simulink model "system_2022 [23-03-03]"  (R2022a)
settings: Solver=FixedStepAuto  StartTime=0.0  StopTime=30  FixedStep=0.05  MinStep=0.01  RelTol=1e-3  EnableMultiTasking=on
libraries: mbedblockslib x24, simulink x6, hdlsllib x6, slpidlib x3
(part 1 of 3)
settings Model: ExtModeTrigDuration=10  Creator=MATLAB  LastModifiedBy=FUGAZI
settings SolverCC: ZeroCrossControl=DisableAll  AutoInsertRateTranBlk=on
settings OptimizationCC: EnhancedBackFolding=on  PassReuseOutputArgsAs=Individual arguments  ZeroExternalMemoryAtStartup=off  ZeroInternalMemoryAtStartup=off  MaxStackSize=64  OptimizeBlockOrder=speed  DifferentSizesBufferReuse=on  OptimizationCustomize=off  EfficientTunableParamExpr=on
settings DebuggingCC: MultiTaskDSMMsg=none  ParameterTunabilityLossMsg=error
settings HardwareCC: ProdBitPerPointer=32  ProdBitPerSizeT=32  ProdBitPerPtrDiffT=32  ProdLargestAtomicInteger=Long  ProdLargestAtomicFloat=Double  ProdWordSize=32  ProdLongLongMode=on  ProdHWDeviceType=ARM Compatible->ARM Cortex
settings SFSimCC: MATLABDynamicMemAlloc=off
settings RTWCC: SystemTargetFile=ert.tlc  HardwareBoard=STM32 Nucleo L476RG  TemplateMakefile=ert_default_tmf  Toolchain=GNU Tools for ARM Embedded Processors
settings CodeAppCC: ForceParamTrailComments=on  IgnoreCustomStorageClasses=off  OperatorAnnotations=on  SimulinkDataObjDesc=on  SFDataObjDesc=on  InsertBlockDesc=on
settings ERTTargetCC: SupportContinuousTime=on  ExtModeTransport=3  ExtModeStaticAlloc=on  ExtModeStaticAllocSize=2000  ExtModeMexFile=ext_xcp  ExtModeIntrfLevel=Level2 - Open

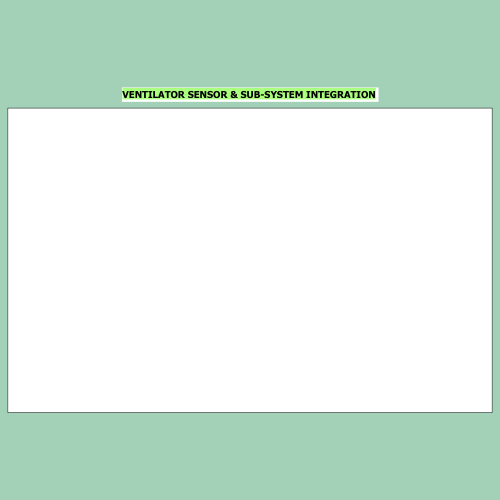
[thumbnail: Simulink's stored preview of the top-level diagram]
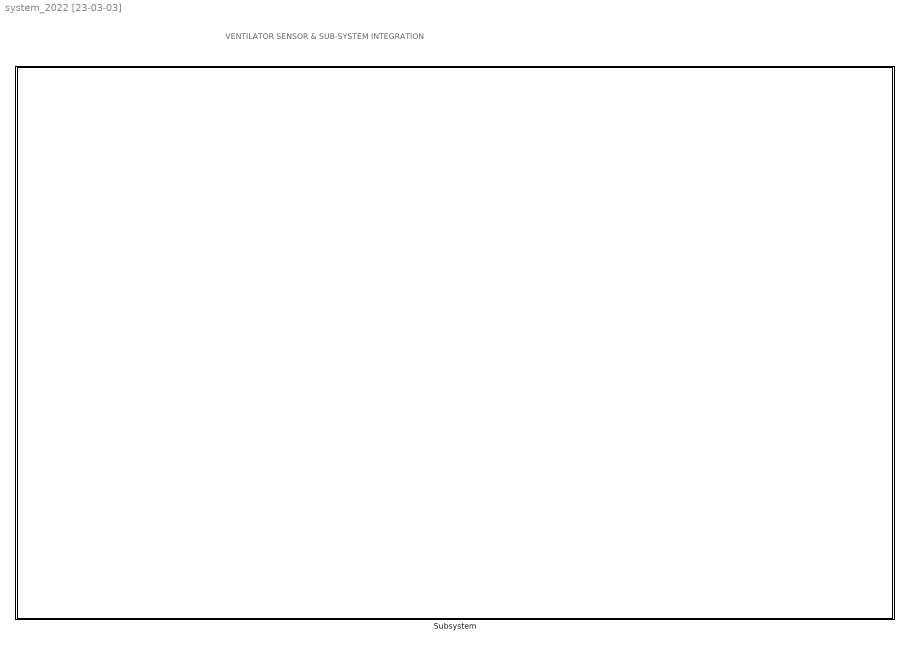
== system system_2022 [23-03-03] ==
  note: VENTILATOR SENSOR & SUB-SYSTEM INTEGRATION
  Subsystem : Subsystem

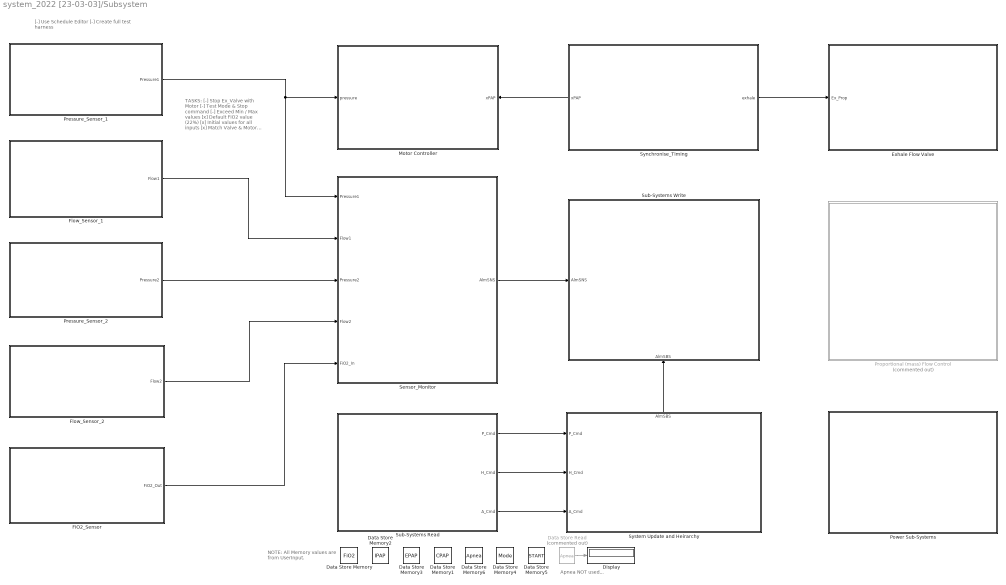
== system system_2022 [23-03-03]/Subsystem ==
  note: Apnea NOT used...
  note: TASKS:
      | [-] Stop Ex_Valve with Motor
      | [-] Test Mode & Stop command
      | [-] Exceed Min / Max values
      | [x] Default FiO2 value (22%)
      | [x] Initial values for all inputs
      | [x] Match Valve & Motor timing
      | [x] Start/Stop bit activate
      | [x] CPAP / BiPAP Mode select
      | [x] Initial CPAP value at boot
  note: [-] Use Schedule Editor
      | [-] Create full test harness
  note: NOTE: All Memory values
      | are from UserInput.
  Data Store Memory : DataStoreMemory  DataStoreName=FiO2  WriteAfterWriteMsg=warning  ShowAdditionalParam=off
  Data Store Memory1 : DataStoreMemory  DataStoreName=CPAP  WriteAfterWriteMsg=warning  ShowAdditionalParam=off
  Data Store Memory2 : DataStoreMemory  DataStoreName=IPAP  WriteAfterWriteMsg=warning  ShowAdditionalParam=off  OutDataTypeStr=uint8
  Data Store Memory3 : DataStoreMemory  DataStoreName=EPAP  WriteAfterWriteMsg=warning  ShowAdditionalParam=off  OutDataTypeStr=uint8
  Data Store Memory4 : DataStoreMemory  DataStoreName=Mode  WriteAfterWriteMsg=warning  ShowAdditionalParam=off
  Data Store Memory5 : DataStoreMemory  DataStoreName=START  WriteAfterWriteMsg=warning  ShowAdditionalParam=off
  Data Store Memory6 : DataStoreMemory  DataStoreName=Apnea  WriteAfterWriteMsg=warning  ShowAdditionalParam=off
  Data Store Read : DataStoreRead  Commented=on  DataStoreName=Apnea  IndexOptions=Index vector (dialog)  Indices=1  OutputSizes=1
  Display : Display
  Exhale Flow Valve : Subsystem
  FiO2_Sensor : Subsystem
  Flow_Sensor_1 : Subsystem
  Flow_Sensor_2 : Subsystem
  Motor Controller : Subsystem
      settings: PortSchema="{\"entries\":[{\"content\":{\"sides\":[{\"content\":{\"connectorIds\":[\"In1\"]},\"type\":\"ConnectorPlacement.EquallySpacedRectSide\",\"uuid\":\"277997a7-2596-41e2-be2a-00a1b5567325\"},{\"content\":{\"connectorIds\":[\"In2\"],\"side\":\"RIGHT\"},\"type\":\"ConnectorPlacement.EquallySpacedRectSide\",\"uuid\":\"4713a00c-a597-4880-a5aa-0886e7233475\"},{\"content\":{\"connectorIds\":[],\"side\":\"TOP\"},\"type\":\"ConnectorPlacement.EquallySpacedRectSide\",\"uuid\":\"80b12314-0e9c-4d27-81c0-11d8cd11bc57\"}]},\"type\":\"ConnectorPlacement.EquallySpacedConnector\",\"uuid\":\"993520d8-11fc-42e6-a5c7-2426b0d2fc8c\"}],\"packageUris\":[\"http://schema.mathworks.com/mf0/Connector/R2020b\"],\"version\":\"1.0\"}"
  Power Sub-Systems : Subsystem
  Pressure_Sensor_1 : Subsystem
  Pressure_Sensor_2 : Subsystem
  Proportional (mass) Flow Control : Subsystem  Commented=on
  Sensor_Monitor : Subsystem
  Sub-Systems Read : Subsystem
  Sub-Systems Write : Subsystem
      settings: PortSchema="{\"entries\":[{\"content\":{\"sides\":[{\"content\":{\"connectorIds\":[\"In1\"]},\"type\":\"ConnectorPlacement.EquallySpacedRectSide\",\"uuid\":\"eb9ce795-de09-4ed2-8806-a61f57f93f9b\"},{\"content\":{\"connectorIds\":[],\"side\":\"RIGHT\"},\"type\":\"ConnectorPlacement.EquallySpacedRectSide\",\"uuid\":\"21aaf935-64f9-4c38-8c94-7e839f5ca388\"},{\"content\":{\"connectorIds\":[],\"side\":\"TOP\"},\"type\":\"ConnectorPlacement.EquallySpacedRectSide\",\"uuid\":\"fc84c7b4-5181-42a5-abd6-ccf02989d3da\"},{\"content\":{\"connectorIds\":[\"In2\"],\"side\":\"BOTTOM\"},\"type\":\"ConnectorPlacement.EquallySpacedRectSide\",\"uuid\":\"3d706466-9673-4870-b51b-d2a0bdd6cb85\"}]},\"type\":\"ConnectorPlacement.EquallySpacedConnector\",\"uuid\":\"29ce5ad0-36e4-4e3a-a6a2-cabe895f2242\"}],\"packageUris\":[\"http://schema.mathworks.com/mf0/Connector/R2020b\"],\"version\":\"1.0\"}"
  Synchronise_Timing : Subsystem
      settings: PortSchema="{\"entries\":[{\"content\":{\"sides\":[{\"content\":{\"connectorIds\":[\"Out2\"]},\"type\":\"ConnectorPlacement.EquallySpacedRectSide\",\"uuid\":\"63dc7675-ee32-444b-9275-4cbd91f7699a\"},{\"content\":{\"connectorIds\":[\"Out1\"],\"side\":\"RIGHT\"},\"type\":\"ConnectorPlacement.EquallySpacedRectSide\",\"uuid\":\"5dbf7e88-4898-4ed4-90a6-8ca6dfa4b96e\"},{\"content\":{\"connectorIds\":[],\"side\":\"TOP\"},\"type\":\"ConnectorPlacement.EquallySpacedRectSide\",\"uuid\":\"7e7cd6c7-7c73-4e47-93fd-71beedff7f82\"}]},\"type\":\"ConnectorPlacement.EquallySpacedConnector\",\"uuid\":\"7bb074e5-16ae-4f8c-9a99-c8e825a4014c\"}],\"packageUris\":[\"http://schema.mathworks.com/mf0/Connector/R2020b\"],\"version\":\"1.0\"}"
  System Update and Heirarchy : Subsystem
      settings: PortSchema="{\"entries\":[{\"content\":{\"sides\":[{\"content\":{\"connectorIds\":[\"In1\",\"In2\",\"In3\"]},\"type\":\"ConnectorPlacement.EquallySpacedRectSide\",\"uuid\":\"2e4a90fa-3ed6-459b-ba0d-351f76e300d2\"},{\"content\":{\"connectorIds\":[],\"side\":\"RIGHT\"},\"type\":\"ConnectorPlacement.EquallySpacedRectSide\",\"uuid\":\"e2fc2115-9220-4948-a1d6-003b6dee47b7\"},{\"content\":{\"connectorIds\":[\"Out1\"],\"side\":\"TOP\"},\"type\":\"ConnectorPlacement.EquallySpacedRectSide\",\"uuid\":\"5feddca4-6301-4c9a-bd70-4ed3ce5f33af\"},{\"content\":{\"connectorIds\":[],\"side\":\"BOTTOM\"},\"type\":\"ConnectorPlacement.EquallySpacedRectSide\",\"uuid\":\"ff07628e-9dd0-4bec-99a6-7b920e9dd097\"}]},\"type\":\"ConnectorPlacement.EquallySpacedConnector\",\"uuid\":\"e118aa99-09e8-4c0c-a1cb-9c50b6e2eab2\"}],\"packageUris\":[\"http://schema.mathworks.com/mf0/Connector/R2020b\"],\"version\":\"1.0\"}"
  wires:
  Pressure_Sensor_1/1(Pressure1) -> Sensor_Monitor/1(Pressure1), Motor Controller/1(pressure)
  FiO2_Sensor/1(FiO2_Out) -> Sensor_Monitor/5(FiO2_In)
  Pressure_Sensor_2/1(Pressure2) -> Sensor_Monitor/3(Pressure2)
  System Update and Heirarchy/1(AlmSBS) -> Sub-Systems Write/2(AlmSBS)
  Sub-Systems Read/3(A_Cmd) -> System Update and Heirarchy/3(A_Cmd)
  Sub-Systems Read/1(P_Cmd) -> System Update and Heirarchy/1(P_Cmd)
  Sensor_Monitor/1(AlmSNS) -> Sub-Systems Write/1(AlmSNS)
  Flow_Sensor_2/1(Flow2) -> Sensor_Monitor/4(Flow2)
  Flow_Sensor_1/1(Flow1) -> Sensor_Monitor/2(Flow1)
  Sub-Systems Read/2(H_Cmd) -> System Update and Heirarchy/2(H_Cmd)
  Synchronise_Timing/2(xPAP) -> Motor Controller/2(xPAP)
  Synchronise_Timing/1(exhale) -> Exhale Flow Valve/1(Ex_Prop)
  Data Store Read/1 -> Display/1

== system system_2022 [23-03-03]/Subsystem/Exhale Flow Valve ==
  note: Value In = % Duty Cycle
  note: How to get varying PWM signal?
  note: Exhalation Proportional Solenoid
  note: Con P11 - Pin 3 & 4
  Ex_Prop : Inport
  Convert to logical : DataTypeConversion  SaturateOnIntegerOverflow=off  RndMeth=Floor
  PWM Output : mbedblockslib/PWM Output  Pin=PA_8  EnableInputFrequency=off  InitialFrequency=500  InitialDutyCycle=85  NotificationType=None
      settings: SourceProductBaseCode=MICROBIT,NUCLEO,STMICRODIS
  Repeating Sequence1 : simulink/Sources/Repeating Sequence  Commented=on  rep_seq_t=[0 1.3 1.4 2.5 2.6]  rep_seq_y=[15 15 71 71 15]
  Scope : Scope
  wires:
  Convert to logical/1 -> PWM Output/1
  Ex_Prop/1 -> Scope/1, Convert to logical/1

== system system_2022 [23-03-03]/Subsystem/FiO2_Sensor ==
  note: Analog READ
  note: READ ADC - FiO2 Sensor
      | Convert to [20%-100%] & update array[4]
  note: FiO2 Trigger Values:
      | 0x71 = 113 - FiO2 Normal
      | 0x72 = 114 - FiO2 Low
      | 0x73 = 115 - FiO2 High
  note: Converted FiO2?
  note: Convert
      | to 5V?
  note: Output: 8 - 13mV
  note: 1023 steps (decimal)
  note: input x (5/1023)
  Analog Input : mbedblockslib/Analog Input  Commented=on  Pin=A0  ReadResultsOnly=off  ConversionTriggerSource=Software  ExternalTriggerType=uint32( 0 )  OutputDataType=double  EnableConversionCompleteNotify=off  EnableOuputStatus=off  SampleTime=-1
      settings: SourceProductBaseCode=MICROBIT,NUCLEO,STMICRODIS
  Constant : Constant  Value=4
  Display : Display
  Display1 : Display
  Display2 : Display
  FiO2 : Constant  Value=9025
  Gain : Gain  Gain=5/1023
  Round : Rounding  Operator=round
  Subsystem2 : Subsystem
  To Percent : Gain  Gain=1/100
  FiO2_Out : Outport
  wires:
  Gain/1 -> Round/1
  Subsystem2/1(Flow2) -> Display2/1
  Constant/1 -> Subsystem2/1(Index1)
  [FLOW_AR2] -> Subsystem2/3(Array)
  FiO2/1 -> Gain/1
  Round/1 -> To Percent/1, Subsystem2/2(Sense1), Display/1
  To Percent/1 -> Display1/1, FiO2_Out/1

== system system_2022 [23-03-03]/Subsystem/Flow_Sensor_1 ==
  note: NO_FLOW = 0x1111 = 237L/m
  note: Unsigned is incorrect?
  note: FLOW_SENSOR_1
      | (I2C_2 READ)
      | READ I2C_2 - SFM3200 Flow Sensor
      | Convert to SLM & update array
  note: Def_Addr = 0x40
      | Read_Addr = 0x81
  note: I2C_2: Flow Sensor
      | SCL_2 = D6
      | SDA_2 = PB_11
  note: I2C_0: Sub-System
      | SCL_0 = D10
      | SDA_0 = PB_7
      | Slave Address: 0X55
  note: WRITE TO HMI
  note: SLM
  note: convert to positive
  note: Update Sensor Array
  note: Flow Rate Range: 10sL/m - 80sL/m
  note: Connector P10
  Abs : Abs  SaturateOnIntegerOverflow=off
  Constant : Constant
  Convert to L/m : Subsystem
  Display : Display
  Display2 : Display
  I2C Convert : Subsystem
  I2C Master Read : mbedblockslib/I2C Master Read  Commented=on  I2CModule=2  Mode=Master  SlaveAddress=hex2dec('81')  SlaveByteOrder=BigEndian  Direction=Receiver  RegisterAddressMode=off  RegisterAddress=uint8(1)  SlaveDataType=uint8  DataLength=2  NoAck=on  RepeatedStart=off  OutputStatus=off  SampleTime=0.1
      settings: SourceProductBaseCode=MICROBIT,NUCLEO,STMICRODIS
  I2C Master Write : mbedblockslib/I2C Master Write  Commented=on  I2CModule=0  Mode=Master  SlaveAddress=uint8(hex2dec('55'))  SlaveByteOrder=BigEndian  Direction=Transmitter  RegisterAddressMode=off  RegisterAddress=uint8(hex2dec('11'))  SlaveDataType=uint8  DataLength=2  NoAck=off  RepeatedStart=off  OutputStatus=off
      settings: SourceProductBaseCode=MICROBIT,NUCLEO,STMICRODIS
  Round1 : Rounding  Operator=round
  Subsystem2 : Subsystem
  Flow1 : Outport
  wires:
  I2C Master Read/1 -> I2C Convert/1(In1)
  I2C Convert/1(Out1) -> Convert to L/m/1(In1)
  Round1/1 -> Abs/1
  Convert to L/m/1(Out1) -> Round1/1
  Constant/1 -> Subsystem2/1(Index1)
  Subsystem2/1(Flow2) -> Display2/1
  [PRES_AR1] -> Subsystem2/3(Array)
  Abs/1 -> Subsystem2/2(Sense1), I2C Master Write/1, Display/1, Flow1/1

== system system_2022 [23-03-03]/Subsystem/Flow_Sensor_2 ==
  note: Flow Trigger Values:
      | 0x61 = 97 - Normal Op
      | 0x62 = 98 - FlowRate2 High
      | 0x63 = 99 - FlowRate2 Low
  note: Converted Flow2
  note: FLOW_SENSOR_2
      | (I2C_2 READ)
      | READ I2C_? - SFM3200 Flow Sensor2
      | Convert to SLM & update array[3]
  note: Def_Addr = 0x40
      | Read_Addr = 0x81
  note: Simulation Value
  note: I2C_0: Flow Sensor
      | (Same as Sub-Systems)
      | SCL_2 = D10
      | SDA_2 = PB_7
  note: convert to positive
  note: Unsigned is incorrect?
  note: Flow Rate Range: 10sL/m - 80sL/m
  note: SLM
  Abs : Abs  SaturateOnIntegerOverflow=off
  Constant : Constant  Value=3
  Display : Display
  Display2 : Display
  I2C Master Read : mbedblockslib/I2C Master Read  Commented=on  I2CModule=2  Mode=Master  SlaveAddress=hex2dec('81')  SlaveByteOrder=BigEndian  Direction=Receiver  RegisterAddressMode=off  RegisterAddress=uint8(1)  SlaveDataType=uint8  DataLength=2  NoAck=on  RepeatedStart=off  OutputStatus=off  SampleTime=0.1
      settings: SourceProductBaseCode=MICROBIT,NUCLEO,STMICRODIS
  Round1 : Rounding  Operator=round
  Subsystem : Subsystem
  Subsystem1 : Subsystem
  Subsystem2 : Subsystem
  Flow2 : Outport
  wires:
  Subsystem2/1(Flow2) -> Display2/1
  Constant/1 -> Subsystem2/1(Index1)
  [PRES_AR2] -> Subsystem2/3(Array)
  I2C Master Read/1 -> Subsystem/1(In1)
  Round1/1 -> Abs/1
  Subsystem/1(Out1) -> Subsystem1/1(In1)
  Subsystem1/1(Out1) -> Round1/1
  Abs/1 -> Subsystem2/2(Sense1), Flow2/1, Display/1

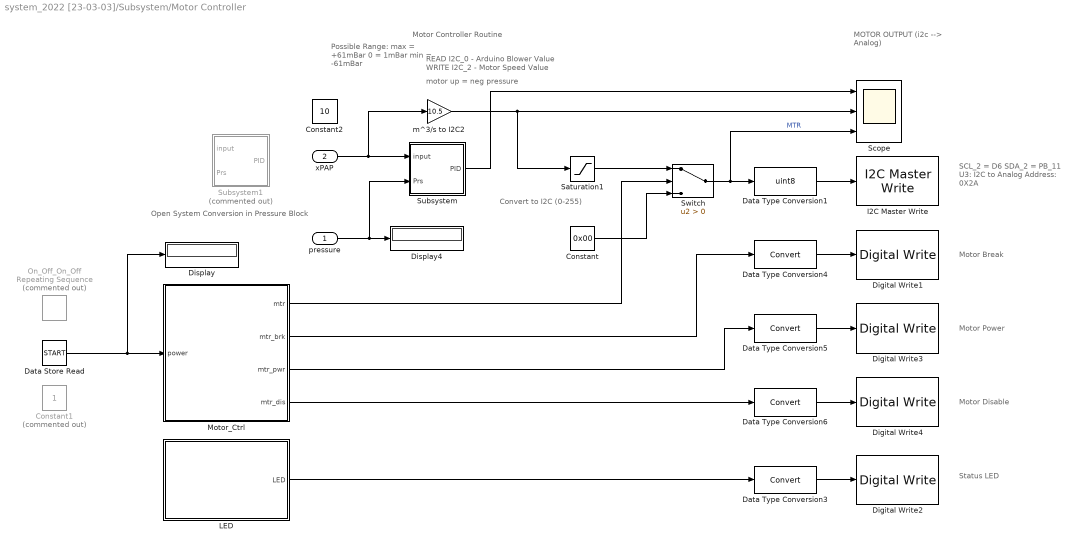
== system system_2022 [23-03-03]/Subsystem/Motor Controller ==
  note: Open System Conversion in Pressure Block
  note: Convert to I2C
      | (0-255)
  note: Motor Controller Routine
  note: motor up = neg pressure
  note: MOTOR OUTPUT
      | (i2c --> Analog)
  note: SCL_2 = D6
      | SDA_2 = PB_11
      | U3: I2C to Analog
      | Address: 0X2A
  note: Motor Break
  note: Motor Power
  note: Motor Disable
  note: Possible Range:
      | max = +61mBar
      | 0 = 1mBar
      | min = -61mBar
  note: READ  I2C_0  - Arduino Blower Value
      | WRITE I2C_2 - Motor Speed Value
  note: Status LED
  pressure : Inport
  xPAP : Inport  Port=2
  Constant : Constant  Value=0x00
  Constant1 : Constant  Commented=on
  Constant2 : Constant  Value=10
  Data Store Read : DataStoreRead  DataStoreName=START  IndexOptions=Index vector (dialog)  Indices=1  OutputSizes=1
  Data Type Conversion1 : DataTypeConversion  OutDataTypeStr=uint8  SaturateOnIntegerOverflow=off  RndMeth=Floor
  Data Type Conversion{3..6} (4 alike) : DataTypeConversion  SaturateOnIntegerOverflow=off  RndMeth=Floor
  Digital Write1 : mbedblockslib/Digital Write  Pin=PC_3  Direction=output
      settings: SourceProductBaseCode=MICROBIT,NUCLEO,STMICRODIS
  Digital Write2 : mbedblockslib/Digital Write  Pin=PB_0  Direction=output
      settings: SourceProductBaseCode=MICROBIT,NUCLEO,STMICRODIS
  Digital Write3 : mbedblockslib/Digital Write  Pin=PB_9  Direction=output
      settings: SourceProductBaseCode=MICROBIT,NUCLEO,STMICRODIS
  Digital Write4 : mbedblockslib/Digital Write  Pin=PC_4  Direction=output
      settings: SourceProductBaseCode=MICROBIT,NUCLEO,STMICRODIS
  Display : Display
  Display4 : Display
  I2C Master Write : mbedblockslib/I2C Master Write  I2CModule=2  Mode=Master  SlaveAddress=uint8(hex2dec('2A'))  SlaveByteOrder=BigEndian  Direction=Transmitter  RegisterAddressMode=on  RegisterAddress=uint8(hex2dec('10'))  SlaveDataType=uint8  DataLength=2  NoAck=off  RepeatedStart=off  OutputStatus=off
      settings: SourceProductBaseCode=MICROBIT,NUCLEO,STMICRODIS
  LED : Stateflow chart  TreatAsAtomicUnit=on
  Motor_Ctrl : Stateflow chart  TreatAsAtomicUnit=on
  On_Off_On_Off : simulink/Sources/Repeating Sequence  Commented=on  rep_seq_t=[0 5 5.05 10 10.05 15 15.05 20]  rep_seq_y=[1 1 0 0 1 1 0 0]
  Saturation1 : Saturate  UpperLimit=255  LowerLimit=0
  Scope : Scope  NumInputPorts=3
  Subsystem : Subsystem
  Subsystem1 : Subsystem  Commented=on
  Switch : Switch  Criteria=u2 > Threshold  SaturateOnIntegerOverflow=off  InputSameDT=off
  m^3/s to I2C2 : Gain  Gain=10.5
  wires:
  Data Type Conversion1/1 -> I2C Master Write/1
  Data Type Conversion5/1 -> Digital Write3/1
  Data Type Conversion4/1 -> Digital Write1/1
  Data Type Conversion6/1 -> Digital Write4/1
  Constant/1 -> Switch/3
  Motor_Ctrl/4(mtr_dis) -> Data Type Conversion6/1
  Motor_Ctrl/3(mtr_pwr) -> Data Type Conversion5/1
  Motor_Ctrl/2(mtr_brk) -> Data Type Conversion4/1
  Data Type Conversion3/1 -> Digital Write2/1
  LED/1(LED) -> Data Type Conversion3/1
  Saturation1/1 -> Switch/1
  Switch/1 -> Scope/3, Data Type Conversion1/1  "MTR"
  Motor_Ctrl/1(mtr) -> Switch/2
  pressure/1 -> Subsystem/2(Prs), Display4/1
  Data Store Read/1 -> Display/1, Motor_Ctrl/1(power)
  xPAP/1 -> Subsystem/1(input), m^3/s to I2C2/1
  m^3/s to I2C2/1 -> Scope/2, Saturation1/1
  Subsystem/1(PID) -> Scope/1

== system system_2022 [23-03-03]/Subsystem/Power Sub-Systems ==
  note: After delay, Switch on Sub-Systems
      | (HMI & ALARM)
  note: HMI Power
      | (6V)
  note: Alarm Power
      | (6V)
  Data Type Conversion1 : DataTypeConversion  SaturateOnIntegerOverflow=off  RndMeth=Floor
  Data Type Conversion3 : DataTypeConversion  SaturateOnIntegerOverflow=off  RndMeth=Floor
  Digital Write1 : mbedblockslib/Digital Write  Pin=PB_4  Direction=output
      settings: SourceProductBaseCode=MICROBIT,NUCLEO,STMICRODIS
  Digital Write2 : mbedblockslib/Digital Write  Pin=PB_5  Direction=output
      settings: SourceProductBaseCode=MICROBIT,NUCLEO,STMICRODIS
  POWER : Stateflow chart  TreatAsAtomicUnit=on
  wires:
  POWER/1(HMI_Pwr) -> Data Type Conversion3/1
  Data Type Conversion3/1 -> Digital Write2/1
  Data Type Conversion1/1 -> Digital Write1/1
  POWER/2(ALRM_Pwr) -> Data Type Conversion1/1

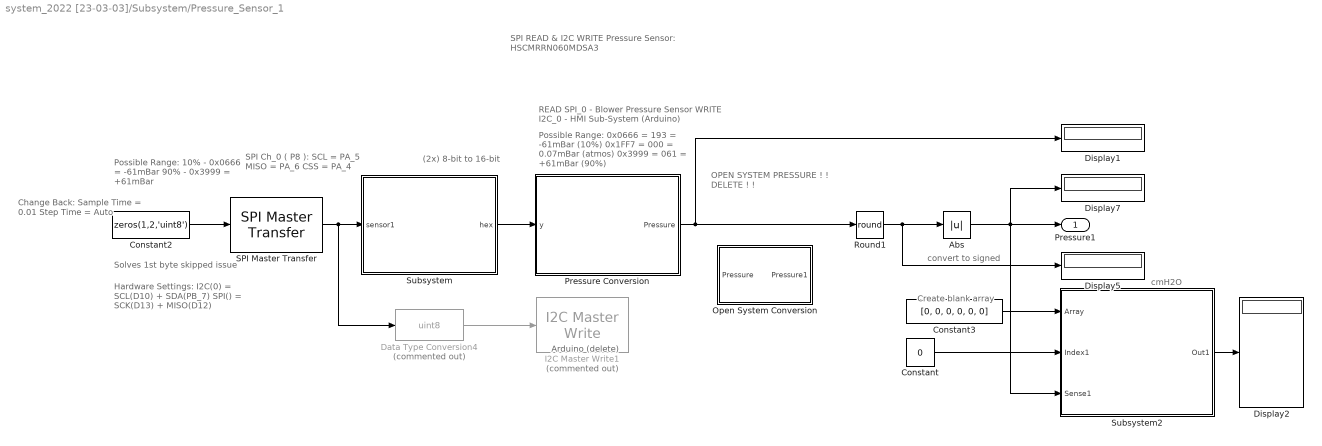
== system system_2022 [23-03-03]/Subsystem/Pressure_Sensor_1 ==
  note: Arduino (delete)
  note: Create blank array
  note: cmH2O
  note: convert to signed
  note: (2x) 8-bit to 16-bit
  note: SPI READ & I2C WRITE
      | Pressure Sensor: HSCMRRN060MDSA3
  note: READ SPI_0  -  Blower Pressure Sensor
      | WRITE I2C_0 - HMI Sub-System (Arduino)
  note: SPI Ch_0 ( P8 ):
      | SCL = PA_5
      | MISO = PA_6
      | CSS = PA_4
  note: Possible Range:
      | 10% - 0x0666 = -61mBar
      | 90% - 0x3999 = +61mBar
  note: Solves 1st byte
      | skipped issue
  note: Possible Range:
      | 0x0666 = 193 = -61mBar (10%)
      | 0x1FF7 = 000 = 0.07mBar (atmos)
      | 0x3999 = 061 = +61mBar (90%)
  note: Hardware Settings:
      | I2C(0) = SCL(D10) + SDA(PB_7)
      | SPI() = SCK(D13) + MISO(D12)
  note: OPEN SYSTEM PRESSURE
      | ! ! DELETE ! !
  note: Change Back:
      | Sample Time = 0.01
      | Step Time = Auto
  Abs : Abs  SaturateOnIntegerOverflow=off
  Constant : Constant  Value=0
  Constant2 : Constant  Value=zeros(1,2,'uint8')  OutDataTypeStr=uint8  SampleTime=0.1
  Constant3 : Constant  Value=[0, 0, 0, 0, 0, 0]
  Data Type Conversion4 : DataTypeConversion  Commented=on  OutDataTypeStr=uint8  SaturateOnIntegerOverflow=off  RndMeth=Floor
  Display{1..2,5,7} (4 alike) : Display
  I2C Master Write1 : mbedblockslib/I2C Master Write  Commented=on  I2CModule=0  Mode=Master  SlaveAddress=uint8(hex2dec('55'))  SlaveByteOrder=BigEndian  Direction=Transmitter  RegisterAddressMode=off  RegisterAddress=uint8(hex2dec('11'))  SlaveDataType=uint8  DataLength=2  NoAck=off  RepeatedStart=off  OutputStatus=off
      settings: SourceProductBaseCode=MICROBIT,NUCLEO,STMICRODIS
  Open System Conversion : Subsystem
  Pressure Conversion : Subsystem
  Round1 : Rounding  Operator=round
  SPI Master Transfer : mbedblockslib/SPI Master Transfer  SPIModule=0  Mode=Master  BusSpeed=uint32( 1000000 )  Pin=PA_4  FirstBitToTransfer=Most significant bit (MSB)  ClockMode=0  BlockFunction=Transfer  RegisterAddress=0  OutputDataType=int8  OutputDataLength=1  UseCustomSSPin=Explicit GPIO calls  ActiveLowSSPin=Active low
      settings: SourceProductBaseCode=MICROBIT,NUCLEO,STMICRODIS
  Subsystem : Subsystem
  Subsystem2 : Subsystem
  Pressure1 : Outport
  wires:
  SPI Master Transfer/1 -> Subsystem/1(sensor1), Data Type Conversion4/1
  Subsystem/1(hex) -> Pressure Conversion/1(y)
  Constant2/1 -> SPI Master Transfer/1
  Round1/1 -> Abs/1, Display5/1
  Constant3/1 -> Subsystem2/1(Array)
  Constant/1 -> Subsystem2/2(Index1)
  Subsystem2/1(Out1) -> Display2/1
  Data Type Conversion4/1 -> I2C Master Write1/1
  Abs/1 -> Subsystem2/3(Sense1), Display7/1, Pressure1/1
  Pressure Conversion/1(Pressure) -> Round1/1, Display1/1

== system system_2022 [23-03-03]/Subsystem/Pressure_Sensor_2 ==
  note: SPI READ
  note: READ SPI_2 - Exhale Pressure Sensor
      | Convert to cmH2O & pass value array
  note: Pressure Range:
      | 0x51 = 81 - Normal Op
      | 0x52 = 82 - Pressure2 High
      | 0x53 = 83 - Pressure 2 Low
  note: Array "From"
  note: SPI Ch_2:
      | CSS = PB_12
      | SCL = PB_13
      | MISO = PB_14
  note: Solves 1st byte
      | skipped issue
  note: (2x) 8-bit to 16-bit
  note: Possible Range:
      | 0x0666 = 193 = -61mBar (10%)
      | 0x1FF7 = 000 = 0.07mBar (atmos)
      | 0x3999 = 061 = +61mBar (90%)
  note: (TEST) Write to HMI
  note: convert to signed
  Abs : Abs  SaturateOnIntegerOverflow=off
  Constant : Constant  Value=2
  Constant2 : Constant  Value=zeros(1,2,'uint8')  OutDataTypeStr=uint8
  Display : Display
  Display2 : Display
  I2C Master Write1 : mbedblockslib/I2C Master Write  Commented=on  I2CModule=0  Mode=Master  SlaveAddress=uint8(hex2dec('55'))  SlaveByteOrder=BigEndian  Direction=Transmitter  RegisterAddressMode=off  RegisterAddress=uint8(hex2dec('11'))  SlaveDataType=uint8  DataLength=2  NoAck=off  RepeatedStart=off  OutputStatus=off
      settings: SourceProductBaseCode=MICROBIT,NUCLEO,STMICRODIS
  Pressure Conversion : Subsystem
  Round1 : Rounding  Operator=round
  SPI Master Transfer : mbedblockslib/SPI Master Transfer  Commented=on  SPIModule=2  Mode=Master  BusSpeed=uint32( 1000000 )  Pin=PB_12  FirstBitToTransfer=Most significant bit (MSB)  ClockMode=0  BlockFunction=Transfer  RegisterAddress=0  OutputDataType=int8  OutputDataLength=1  UseCustomSSPin=Explicit GPIO calls  ActiveLowSSPin=Active low
      settings: SourceProductBaseCode=MICROBIT,NUCLEO,STMICRODIS
  Subsystem : Subsystem
  Subsystem2 : Subsystem
  Pressure2 : Outport
  wires:
  Constant/1 -> Subsystem2/1(Index1)
  Subsystem2/1(Flow2) -> Display2/1
  [FLOW_AR1] -> Subsystem2/3(Array)
  Constant2/1 -> SPI Master Transfer/1
  Pressure Conversion/1(Pressure) -> Round1/1
  Subsystem/1(hex) -> Pressure Conversion/1(y)
  SPI Master Transfer/1 -> I2C Master Write1/1, Subsystem/1(sensor1)
  Abs/1 -> Subsystem2/2(Sense1), Pressure2/1, Display/1
  Round1/1 -> Abs/1

== system system_2022 [23-03-03]/Subsystem/Proportional (mass) Flow Control ==
  note: Check power supply = 24V
  note: Already in %
  note: Mass Flow Controller (MFC) Valve
      | STM32: Master_I2C to I2C_DAC
  note: U3: I2C to Analog
      | SCL_2 = D6
      | SDA_2 = PB_11
      | Slave Address: 0X2A
      | Register Adress_1: 0x10
      | Register Adress_2: 0x11
  note: STM32 - I2C - DAC - Analog_Amp - 4-20mA - Prop_Flow (Type 8741)
  note: Control Pins:
      | (out) Dig_In =
      | (out) Rel_NC =
      | (in) Prop_Fl =
  note: FiO2 User %
  note: FiO2 sensor %
  note: I2C control range: 0x-- - 0x--?
      | Convert to smaller range
  note: Already in %
  Constant : Constant  Value=0.44
  Data Store Read : DataStoreRead  DataStoreName=FiO2  IndexOptions=Index vector (dialog)  Indices=1  OutputSizes=1
  Data Type Conversion1 : DataTypeConversion  OutDataTypeStr=uint8  SaturateOnIntegerOverflow=off  RndMeth=Floor
  Discrete PID Controller1 : slpidlib/PID Controller  Controller=PID  Form=Parallel  TimeDomain=Discrete-time  UseExternalTs=off  SampleTime=0.001  IntegratorMethod=Forward Euler  FilterMethod=Forward Euler  ControllerParametersSource=internal  P=5  I=5  UseKiTs=on  D=10  N=180  UseFilter=on  TunerSelectOption=Transfer Function Based (PID Tuner App)  InitialConditionSource=internal  InitialConditionForIntegrator=0  InitialConditionForFilter=0  DifferentiatorICPrevScaledInput=0  ExternalReset=none  TrackingMode=off  Kt=1  LimitOutput=on  SatLimitsSource=internal  UpperSaturationLimit=22  LowerSaturationLimit=0  LinearizeAsGain=off  AntiWindupMode=none  Kb=1  POutMin=[]  POutMax=[]  IOutMin=[]  IOutMax=[]  DOutMin=[]  DOutMax=[]  NOutMin=[]  NOutMax=[]  SumOutMin=[]  SumOutMax=[]  SaturationOutMin=[]  SaturationOutMax=[]  PParamMin=[]  PParamMax=[]  IParamMin=[]  IParamMax=[]  DParamMin=[]  DParamMax=[]  NParamMin=[]  NParamMax=[]  KbParamMin=[]  KbParamMax=[]  KtParamMin=[]  KtParamMax=[]  KbOutMin=[]  KbOutMax=[]  KtOutMin=[]  KtOutMax=[]  IntegratorOutMin=[]  IntegratorOutMax=[]  FilterOutMin=[]  FilterOutMax=[]  SumI1OutMin=[]  SumI1OutMax=[]  SumI2OutMin=[]  SumI2OutMax=[]  SumI3OutMin=[]  SumI3OutMax=[]  SumI4OutMin=[]  SumI4OutMax=[]  SumDOutMin=[]  SumDOutMax=[]  DifferentiatorOutMin=[]  DifferentiatorOutMax=[]  FilterDiffOutCoefMin=[]  FilterDiffOutCoefMax=[]  ReciprocalOutMin=[]  ReciprocalOutMax=[]  SumDenOutMin=[]  SumDenOutMax=[]  SumNumOutMin=[]  SumNumOutMax=[]  DivideOutMin=[]  DivideOutMax=[]  UdiffTsProdOutMin=[]  UdiffTsProdOutMax=[]  NTsProdOutMin=[]  NTsProdOutMax=[]  UintegralTsProdOutMin=[]  UintegralTsProdOutMax=[]  UngainTsProdOutMin=[]  UngainTsProdOutMax=[]  IntegratorContinuousStateAttributes=''  IntegratorStateMustResolveToSignalObject=off  IntegratorRTWStateStorageClass=Auto  FilterContinuousStateAttributes=''  FilterStateMustResolveToSignalObject=off  FilterRTWStateStorageClass=Auto  ParallelPVariant=InternalParameters  IdealPVariant=Disabled  IVariant=InternalParameters  DVariant=InternalParameters  IntegratorVariant=Discrete  SatVariant=Enabled  AWVariant=Passthrough  PCopyVariant=Disabled  TRVariant=Disabled  FdbkBlocksVariant=Forward  IdealPFdbkVariant=Disabled  SatFdbkVariant=Disabled  DerivativeFilterVariant=ForwardEulerFilter  NVariant=InternalParameters  NCopyVariant=Disabled  FilterICVariant=InternalICsFilter  IntegratorICVariant=InternalICs  ExternalResetVariant=Disabled  TRSumVariant=Passthrough  SumFdbkVariant=Disabled  SumVariant=Sum_PID  TsampFilterVariant=InternalTs  TsampNgainVariant=Passthrough  TsampIntegralVariant=Passthrough  ExternalSaturationOutDataTypeStr=Inherit: Same as second input  aMode=0
  Display : Display
  Display1 : Display
  Fraction to FiO2% : Gain  Gain=100
  I2C Master Write : mbedblockslib/I2C Master Write  I2CModule=2  Mode=Master  SlaveAddress=uint8(hex2dec('2A'))  SlaveByteOrder=BigEndian  Direction=Transmitter  RegisterAddressMode=on  RegisterAddress=uint8(hex2dec('11'))  SlaveDataType=uint8  DataLength=2  NoAck=off  RepeatedStart=off  OutputStatus=off
      settings: SourceProductBaseCode=MICROBIT,NUCLEO,STMICRODIS
  Saturation1 : Saturate  UpperLimit=255  LowerLimit=0
  Scope : Scope
  Sum : Sum  Inputs=|+-
  wires:
  Saturation1/1 -> Scope/1, Data Type Conversion1/1
  Data Type Conversion1/1 -> I2C Master Write/1  "SIG"
  Sum/1 -> Discrete PID Controller1/1  "Error"
  Constant/1 -> Sum/1
  Fraction to FiO2%/1 -> Saturation1/1
  [FiO2_out] -> Display1/1
  Discrete PID Controller1/1 -> Fraction to FiO2%/1  "PID"
  Data Store Read/1 -> Display/1, Sum/2

== system system_2022 [23-03-03]/Subsystem/Sensor_Monitor ==
  note: Checks each Sensor's actual value
      | Tragger ALARM value if outside Range
  note: Check for Sensor Alerts & Merge to Single Alarm
  note: 81 = normal
  note: Range Alerts:
      | 0x32 - Pressure1 High
      | 0x33 - Pressure1 Low
      | 0x42 - FlowRate1 High
      | 0x43 - FlowRate1 Low
      | Simulated:
      | 0x52 - Pressure2 High
      | 0x53 - Pressure2 Low
      | 0x62 - FlowRate2 High
      | 0x63 - FlowRate2 Low
      | 0x72 - FiO2 Low
      | 0x73 - FiO2 High
  note: Pressure Sensor
  note: Flow Sensor
  note: 97 = normal
  note: 113 = normal
  note: FiO2 Sensor: 21% - 100%
  note: Flow2 Trigger Values:
      | 0x61 = 97 - Normal Op
      | 0x62 = 98 - FlowRate2 High
      | 0x63 = 99 - FlowRate2 Low
  note: FiO2 Triggers:
      | 0x71 = 113 - Normal Op
      | 0x72 = 114 - FlowRate2 High
      | 0x73 = 115 - FlowRate2 Low
  note: Pressure2 Triggers:
      | 0x51 = 81 - Normal Op
      | 0x52 = 82 - FlowRate2 High
      | 0x53 = 83 - FlowRate2 Low
  note: Flow Sensors:
      | 10sL/m - 80sL/m
  note: Press. Sensor:
      | 5 - 20 cmH2O
  note: Flow1 Trigger Values:
      | 0x41 = 65 - Normal Op
      | 0x42 = 66 - FlowRate2 High
      | 0x43 = 67 - FlowRate2 Low
  note: Pressure1 Triggers:
      | 0x31 = 49 - Normal Op
      | 0x32 = 50 - FlowRate2 High
      | 0x33 = 51 - FlowRate2 Low
  note: Press. Sensor:
      | 5 - 20 cmH2O
  note: Flow Sensors:
      | 10sL/m - 80sL/m
  Pressure1 : Inport
  Flow1 : Inport  Port=2
  Pressure2 : Inport  Port=3
  Flow2 : Inport  Port=4
  FiO2_In : Inport  Port=5
  Display : Display
  Display2 : Display
  Flow1_Monitor : Subsystem
  Flow2_Monitor : Subsystem
  Pressure1_Monitor : Subsystem
  Pressure2_Monitor : Subsystem
  Subsystem : Subsystem
      settings: PortSchema="{\"entries\":[{\"content\":{\"sides\":[{\"content\":{\"connectorIds\":[\"In1\",\"In2\"]},\"type\":\"ConnectorPlacement.EquallySpacedRectSide\",\"uuid\":\"974015e2-b79c-4a2c-a375-b0b91b3e2c4e\"},{\"content\":{\"connectorIds\":[\"Out1\"],\"side\":\"RIGHT\"},\"type\":\"ConnectorPlacement.EquallySpacedRectSide\",\"uuid\":\"2b45a403-b560-4258-8fd8-998f3ddc6c2d\"},{\"content\":{\"connectorIds\":[],\"side\":\"TOP\"},\"type\":\"ConnectorPlacement.EquallySpacedRectSide\",\"uuid\":\"5e2dfeab-ffcf-41c7-86c5-27a0241975a3\"},{\"content\":{\"connectorIds\":[\"In3\",\"In4\",\"In5\"],\"side\":\"BOTTOM\"},\"type\":\"ConnectorPlacement.EquallySpacedRectSide\",\"uuid\":\"98c396b8-bf45-4dff-9bbf-be14acd0f892\"}]},\"type\":\"ConnectorPlacement.EquallySpacedConnector\",\"uuid\":\"9a75b7a9-2d56-4c95-810f-4bb7e69b4571\"}],\"packageUris\":[\"http://schema.mathworks.com/mf0/Connector/R2020b\"],\"version\":\"1.0\"}"
  AlmSNS : Outport
  tag scope: FiO2_out=global
  wires:
  Pressure1/1 -> Pressure1_Monitor/1(Pr_I1)
  Flow1/1 -> Flow1_Monitor/1(Flow1)
  Subsystem/1(ALRM_Out) -> Display2/1, AlmSNS/1
  Pressure1_Monitor/1(Pr1_Alrm) -> Subsystem/1(Pr1_Alrm)
  Flow1_Monitor/1(Fl1_Alrm) -> Subsystem/2(Fl1_Alrm)
  FiO2_In/1 -> Display/1, Subsystem/5(Fi_Alrm), [FiO2_out]
  Flow2_Monitor/1(Fl2_Alrm) -> Subsystem/4(Fl2_Alrm)
  Pressure2_Monitor/1(Pr2_Alrm) -> Subsystem/3(Pr2_Alrm)
  Pressure2/1 -> Pressure2_Monitor/1(Pr_E2)
  Flow2/1 -> Flow2_Monitor/1(Flow2)

== system system_2022 [23-03-03]/Subsystem/Sub-Systems Read ==
  note: 0x53 (83) - Trigger
  note: Ignores all 2nd bytes unless
      | User_Input code received
  note: Relay PSU Code to Alarm & HMI
  note: PSU Read
  note: HMI - USER INPUTS:
      | 0x03 (03) - CPAP
      | 0x13 (19) - EPAP
      | 0x23 (35) - IPAP
      | 0x33 (51) - FiO2
      | 0x43 (67) - APNEA
  note: ALARM Responses:
      | 0x21 - Normal Operation
      | 0x22 - Alarm Time_Out (2min)
      | 0x23 - Others ?
  note: ALRM Read
  note: HMI Read
      | I2C(0) = SCL(D10) + SDA(PB_7)
  note: 1st byte = User Input trigger + Which value
      | 2nd byte = Actual value to update system with
  note: PSU Alerts:
      | 0x11 - Normal (AC)
      | 0x12 - Battery 75%
      | 0x13 - Battery 50%
      | 0x14 - Battery 25%
  note: Relay 'snooze' Alarm
  note: Should not receive triggers at the
      | same time (due to series writes)?
  note: HMI ALERTS:
      | 0x01 - Normal (Start/Stop)
      | 0x03 - User_Input (Top_1-5)
      | 0x05 - Alarm (Set/Clear)
      | 0x09 - Mode (Top_0-2)
  note: TESTED
  note: Requires (once-off) boot-up 'initial-values' for each that match HMI initial-values
  note: TESTED
  note: TESTED
  note: Only recieve from Alarm for " Check-Sum"
  Constant : Constant  Value=0x11
  Constant1 : Constant  Value=0x21
  Display : Display
  HMI_Read : mbedblockslib/I2C Master Read  Commented=on  I2CModule=0  Mode=Master  SlaveAddress=hex2dec('55')  SlaveByteOrder=BigEndian  Direction=Receiver  RegisterAddressMode=off  RegisterAddress=uint8(1)  SlaveDataType=uint8  DataLength=2  NoAck=off  RepeatedStart=off  OutputStatus=off  SampleTime=-1
      settings: SourceProductBaseCode=MICROBIT,NUCLEO,STMICRODIS
  HMI_Read1 : mbedblockslib/I2C Master Read  Commented=on  I2CModule=0  Mode=Master  SlaveAddress=hex2dec('10')  SlaveByteOrder=BigEndian  Direction=Receiver  RegisterAddressMode=off  RegisterAddress=uint8(1)  SlaveDataType=uint8  DataLength=2  NoAck=off  RepeatedStart=off  OutputStatus=off  SampleTime=-1
      settings: SourceProductBaseCode=MICROBIT,NUCLEO,STMICRODIS
  HMI_Read2 : mbedblockslib/I2C Master Read  Commented=on  I2CModule=0  Mode=Master  SlaveAddress=hex2dec('15')  SlaveByteOrder=BigEndian  Direction=Receiver  RegisterAddressMode=off  RegisterAddress=uint8(1)  SlaveDataType=uint8  DataLength=2  NoAck=off  RepeatedStart=off  OutputStatus=off  SampleTime=-1
      settings: SourceProductBaseCode=MICROBIT,NUCLEO,STMICRODIS
  HMI_Test_Input : Subsystem
  P_Cmd : Outport
  H_Cmd : Outport  Port=2
  A_Cmd : Outport  Port=3
  wires:
  Constant/1 -> P_Cmd/1
  Constant1/1 -> A_Cmd/1
  HMI_Test_Input/1(H_Cmd) -> Display/1, H_Cmd/1

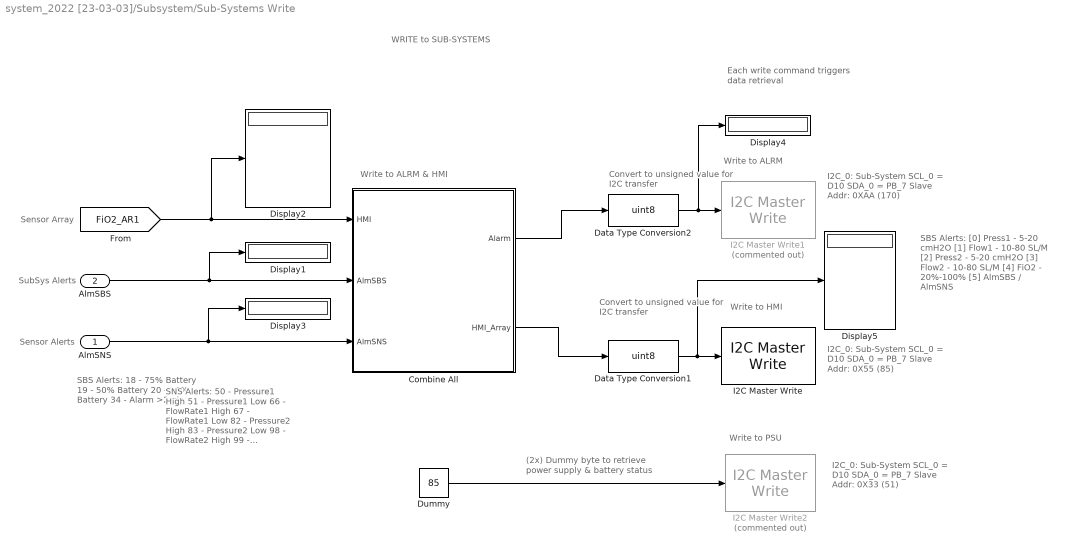
== system system_2022 [23-03-03]/Subsystem/Sub-Systems Write ==
  note: WRITE to SUB-SYSTEMS
  note: SBS Alerts:
      | 18 - 75% Battery
      | 19 - 50% Battery
      | 20 - 25% Battery
      | 34 - Alarm >2min
  note: Write to HMI
  note: Convert to unsigned
      | value for I2C transfer
  note: I2C_0: Sub-System
      | SCL_0 = D10
      | SDA_0 = PB_7
      | Slave Addr: 0X55 (85)
  note: Write to ALRM
  note: I2C_0: Sub-System
      | SCL_0 = D10
      | SDA_0 = PB_7
      | Slave Addr: 0XAA (170)
  note: Convert to unsigned
      | value for I2C transfer
  note: Write to PSU
  note: (2x) Dummy byte to retrieve
      | power supply & battery status
  note: I2C_0: Sub-System
      | SCL_0 = D10
      | SDA_0 = PB_7
      | Slave Addr: 0X33 (51)
  note: Each write command
      | triggers data retrieval
  note: Sensor Alerts
  note: SubSys Alerts
  note: Write to ALRM & HMI
  note: Sensor Array
  note: SBS Alerts:
      | [0] Press1 - 5-20 cmH2O
      | [1] Flow1 - 10-80 SL/M
      | [2] Press2 - 5-20 cmH2O
      | [3] Flow2 - 10-80 SL/M
      | [4] FiO2 - 20%-100%
      | [5] AlmSBS / AlmSNS
  note: SNS Alerts:
      | 50 - Pressure1 High
      | 51 - Pressure1 Low
      | 66 - FlowRate1 High
      | 67 - FlowRate1 Low
      | 82 - Pressure2 High
      | 83 - Pressure2 Low
      | 98 - FlowRate2 High
      | 99 - FlowRate2 Low
      | 114 - FiO2 High
      | 115 - FiO2 Low
  AlmSNS : Inport
  AlmSBS : Inport  Port=2
  Combine All : Subsystem
  Data Type Conversion1 : DataTypeConversion  OutDataTypeStr=uint8  SaturateOnIntegerOverflow=off  RndMeth=Floor
  Data Type Conversion2 : DataTypeConversion  OutDataTypeStr=uint8  SaturateOnIntegerOverflow=off  RndMeth=Floor
  Display{1..5} (5 alike) : Display
  Dummy : Constant  Value=85
  I2C Master Write : mbedblockslib/I2C Master Write  I2CModule=0  Mode=Master  SlaveAddress=uint8(hex2dec('55'))  SlaveByteOrder=BigEndian  Direction=Transmitter  RegisterAddressMode=off  RegisterAddress=uint8(hex2dec('11'))  SlaveDataType=uint8  DataLength=2  NoAck=off  RepeatedStart=off  OutputStatus=off
      settings: SourceProductBaseCode=MICROBIT,NUCLEO,STMICRODIS
  I2C Master Write1 : mbedblockslib/I2C Master Write  Commented=on  I2CModule=0  Mode=Master  SlaveAddress=uint8(hex2dec('AA'))  SlaveByteOrder=BigEndian  Direction=Transmitter  RegisterAddressMode=off  RegisterAddress=uint8(hex2dec('11'))  SlaveDataType=uint8  DataLength=2  NoAck=off  RepeatedStart=off  OutputStatus=off
      settings: SourceProductBaseCode=MICROBIT,NUCLEO,STMICRODIS
  I2C Master Write2 : mbedblockslib/I2C Master Write  Commented=on  I2CModule=0  Mode=Master  SlaveAddress=uint8(hex2dec('33'))  SlaveByteOrder=BigEndian  Direction=Transmitter  RegisterAddressMode=off  RegisterAddress=uint8(hex2dec('11'))  SlaveDataType=uint8  DataLength=2  NoAck=off  RepeatedStart=off  OutputStatus=off
      settings: SourceProductBaseCode=MICROBIT,NUCLEO,STMICRODIS
  wires:
  Data Type Conversion1/1 -> I2C Master Write/1, Display5/1
  Data Type Conversion2/1 -> Display4/1, I2C Master Write1/1
  Dummy/1 -> I2C Master Write2/1
  AlmSNS/1 -> Display3/1, Combine All/3(AlmSNS)
  [FiO2_AR1] -> Combine All/1(HMI), Display2/1
  AlmSBS/1 -> Display1/1, Combine All/2(AlmSBS)
  Combine All/1(Alarm) -> Data Type Conversion2/1
  Combine All/2(HMI_Array) -> Data Type Conversion1/1

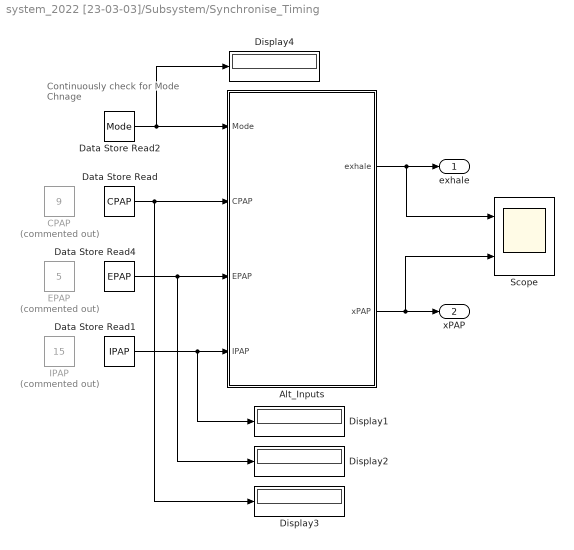
== system system_2022 [23-03-03]/Subsystem/Synchronise_Timing ==
  note: Continuously check
      | for Mode Chnage
  Alt_Inputs : Stateflow chart  TreatAsAtomicUnit=on
  CPAP : Constant  Commented=on  Value=9
  Data Store Read : DataStoreRead  DataStoreName=CPAP  IndexOptions=Index vector (dialog)  Indices=1  OutputSizes=1
  Data Store Read1 : DataStoreRead  DataStoreName=IPAP  DataStoreElements=IPAP  IndexOptions=Index vector (dialog)  Indices=1  OutputSizes=1
  Data Store Read2 : DataStoreRead  DataStoreName=Mode  IndexOptions=Index vector (dialog)  Indices=1  OutputSizes=1
  Data Store Read4 : DataStoreRead  DataStoreName=EPAP  DataStoreElements=EPAP  IndexOptions=Index vector (dialog)  Indices=1  OutputSizes=1
  Display{1..4} (4 alike) : Display
  EPAP : Constant  Commented=on  Value=5
  IPAP : Constant  Commented=on  Value=15
  Scope : Scope  NumInputPorts=2
  exhale : Outport
  xPAP : Outport  Port=2
  wires:
  Alt_Inputs/1(exhale) -> Scope/1, exhale/1
  Alt_Inputs/2(xPAP) -> Scope/2, xPAP/1
  Data Store Read1/1 -> Display1/1, Alt_Inputs/4(IPAP)
  Data Store Read4/1 -> Display2/1, Alt_Inputs/3(EPAP)
  Data Store Read/1 -> Display3/1, Alt_Inputs/2(CPAP)
  Data Store Read2/1 -> Display4/1, Alt_Inputs/1(Mode)

== system system_2022 [23-03-03]/Subsystem/System Update and Heirarchy ==
  note: Store new value accordingly
  note: Check command
      | (upper & lower)
  note: Check Incoming Messages for Alerts/Changes
  note: Pass value to HMI & ALRM (I2C)
  note: Possible Outputs:
      | 0x11 - Normal (AC)
      | 0x12 - Battery 75%
      | 0x13 - Battery 50%
      | 0x14 - Battery 25%
      | 0x21 - No Alarm
      | 0x22 - Alrm Over 2min
  note: Pass value to HMI (I2C)
  note: PSU Cmd Byte
  note: ALRM Cmd Byte
  note: HMI Cmd Byte
  P_Cmd : Inport
  H_Cmd : Inport  Port=2
  A_Cmd : Inport  Port=3
  Alarm Priority : Subsystem
  Display{,1..3} (4 alike) : Display
  Get Value and Array Index : Subsystem
  Initial IPAP EPAP : Subsystem
  Power_CMD : Subsystem
  Update Internal Variables : Subsystem
  AlmSBS : Outport
  wires:
  A_Cmd/1 -> Display1/1, Alarm Priority/2(A_Alrm)
  Alarm Priority/1(ALRM_Out) -> AlmSBS/1
  P_Cmd/1 -> Power_CMD/1(P_Cmd)
  Power_CMD/1(P_Alrm) -> Display3/1, Alarm Priority/1(P_Alrm)
  Get Value and Array Index/2(New_Val1) -> Update Internal Variables/2(New_Val1)
  Get Value and Array Index/1(HMI_Cmd1) -> Update Internal Variables/1(HMI_Cmd1)
  Initial IPAP EPAP/1(output) -> Get Value and Array Index/1(Usr_In), Display/1
  H_Cmd/1 -> Display2/1, Initial IPAP EPAP/1(H_Cmd)

== system system_2022 [23-03-03]/Subsystem/FiO2_Sensor/Subsystem2 ==
  note: Update single element of input array
  Index1 : Inport
  Sense1 : Inport  Port=2
  Array : Inport  Port=3
  Assignment : Assignment  IndexMode=Zero-based  DiagnosticForDimensions=Warning  IndexOptions=Index vector (port)  Indices=0  OutputSizes=1
  Flow2 : Outport
  tag scope: FiO2_AR1=global
  wires:
  Index1/1 -> Assignment/3
  Sense1/1 -> Assignment/2
  Assignment/1 -> [FiO2_AR1], Flow2/1
  Array/1 -> Assignment/1

== system system_2022 [23-03-03]/Subsystem/Flow_Sensor_1/Convert to L//m ==
  note: SLM: Standard Litres pre Minute
  note: Convert to Litres/Min (SLM)
  note: Offset Flow = 0x800
      | Scale Factor = 120
  In1 : Inport
  Constant : Constant  Value=32768
  Constant1 : Constant  Value=0x1111
  Constant2 : Constant  Value=120
  Display : Display
  Divide : Product  Inputs=*/
  Subtract : Sum  Inputs=+-
  Out1 : Outport
  wires:
  Divide/1 -> Display/1, Out1/1
  Subtract/1 -> Divide/1
  Constant2/1 -> Divide/2
  Constant/1 -> Subtract/2
  In1/1 -> Subtract/1

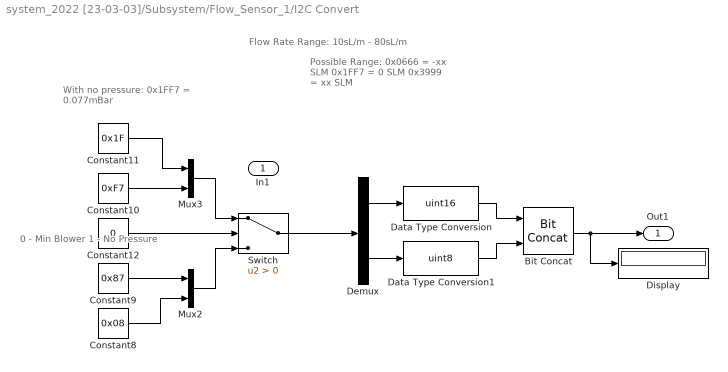
== system system_2022 [23-03-03]/Subsystem/Flow_Sensor_1/I2C Convert ==
  note: Possible Range:
      | 0x0666 = -xx SLM
      | 0x1FF7 = 0 SLM
      | 0x3999 = xx SLM
  note: With no pressure:
      | 0x1FF7 = 0.077mBar
  note: 0 - Min Blower
      | 1 - No Pressure
  note: Flow Rate Range: 10sL/m - 80sL/m
  In1 : Inport
  Bit Concat : hdlsllib/Logic and Bit Operations/Bit Concat  numInputs=2
  Constant10 : Constant  Value=0xF7
  Constant11 : Constant  Value=0x1F
  Constant12 : Constant  Value=0
  Constant8 : Constant  Value=0x08
  Constant9 : Constant  Value=0x87
  Data Type Conversion : DataTypeConversion  OutDataTypeStr=uint16  SaturateOnIntegerOverflow=off  RndMeth=Floor
  Data Type Conversion1 : DataTypeConversion  OutDataTypeStr=uint8  SaturateOnIntegerOverflow=off  RndMeth=Floor
  Demux : Demux  Outputs=2
  Display : Display
      settings: Format=hex (Stored Integer)
  Mux2 : Mux  Inputs=2
  Mux3 : Mux  Inputs=2
  Switch : Switch  Criteria=u2 > Threshold  SaturateOnIntegerOverflow=off  InputSameDT=off
  Out1 : Outport
  wires:
  Data Type Conversion1/1 -> Bit Concat/2
  Bit Concat/1 -> Out1/1, Display/1
  Demux/1 -> Data Type Conversion/1
  Data Type Conversion/1 -> Bit Concat/1
  Demux/2 -> Data Type Conversion1/1
  Constant10/1 -> Mux3/2
  Mux3/1 -> Switch/1
  Mux2/1 -> Switch/3
  Constant9/1 -> Mux2/1
  Constant8/1 -> Mux2/2
  Constant11/1 -> Mux3/1
  Constant12/1 -> Switch/2
  Switch/1 -> Demux/1

== system system_2022 [23-03-03]/Subsystem/Flow_Sensor_1/Subsystem2 ==
  note: Need Global Array??
  note: Update single element of input array
  Index1 : Inport
  Sense1 : Inport  Port=2
  Array : Inport  Port=3
  Assignment : Assignment  IndexMode=Zero-based  DiagnosticForDimensions=Warning  IndexOptions=Index vector (port)  Indices=0  OutputSizes=1
  Flow2 : Outport
  tag scope: FLOW_AR1=global
  wires:
  Index1/1 -> Assignment/3
  Sense1/1 -> Assignment/2
  Assignment/1 -> [FLOW_AR1], Flow2/1
  Array/1 -> Assignment/1

== system system_2022 [23-03-03]/Subsystem/Flow_Sensor_2/Subsystem ==
  note: Possible Range:
      | 0x0666 = -xx SLM
      | 0x1FF7 = 0 SLM
      | 0x3999 = xx SLM
  note: With no pressure:
      | 0x1FF7 = 0.077mBar
  note: 0 - Min Blower
      | 1 - No Pressure
  In1 : Inport
  Bit Concat : hdlsllib/Logic and Bit Operations/Bit Concat  numInputs=2
  Constant10 : Constant  Value=0xF7
  Constant11 : Constant  Value=0x1F
  Constant12 : Constant  Value=0
  Constant8 : Constant  Value=0x70
  Constant9 : Constant  Value=0x97
  Data Type Conversion : DataTypeConversion  OutDataTypeStr=uint16  SaturateOnIntegerOverflow=off  RndMeth=Floor
  Data Type Conversion1 : DataTypeConversion  OutDataTypeStr=uint8  SaturateOnIntegerOverflow=off  RndMeth=Floor
  Demux : Demux  Outputs=2
  Display : Display
      settings: Format=hex (Stored Integer)
  Mux2 : Mux  Inputs=2
  Mux3 : Mux  Inputs=2
  Switch : Switch  Criteria=u2 > Threshold  SaturateOnIntegerOverflow=off  InputSameDT=off
  Out1 : Outport
  wires:
  Data Type Conversion1/1 -> Bit Concat/2
  Bit Concat/1 -> Out1/1, Display/1
  Demux/1 -> Data Type Conversion/1
  Data Type Conversion/1 -> Bit Concat/1
  Demux/2 -> Data Type Conversion1/1
  Constant10/1 -> Mux3/2
  Mux3/1 -> Switch/1
  Mux2/1 -> Switch/3
  Constant9/1 -> Mux2/1
  Constant8/1 -> Mux2/2
  Constant11/1 -> Mux3/1
  Constant12/1 -> Switch/2
  Switch/1 -> Demux/1

== system system_2022 [23-03-03]/Subsystem/Flow_Sensor_2/Subsystem1 ==
  note: SLM: Standard Litres pre Minute
  note: Convert to Litres/Min (SLM)
  note: Offset Flow = 0x800
      | Scale Factor = 120
  In1 : Inport
  Constant : Constant  Value=32768
  Constant2 : Constant  Value=120
  Display : Display
  Divide : Product  Inputs=*/
  Subtract : Sum  Inputs=+-
  Out1 : Outport
  wires:
  Divide/1 -> Display/1, Out1/1
  Subtract/1 -> Divide/1
  Constant2/1 -> Divide/2
  Constant/1 -> Subtract/2
  In1/1 -> Subtract/1

== system system_2022 [23-03-03]/Subsystem/Flow_Sensor_2/Subsystem2 ==
  note: Update single element of input array
  Index1 : Inport
  Sense1 : Inport  Port=2
  Array : Inport  Port=3
  Assignment : Assignment  IndexMode=Zero-based  DiagnosticForDimensions=Warning  IndexOptions=Index vector (port)  Indices=0  OutputSizes=1
  Flow2 : Outport
  tag scope: FLOW_AR2=global
  wires:
  Index1/1 -> Assignment/3
  Sense1/1 -> Assignment/2
  Assignment/1 -> [FLOW_AR2], Flow2/1
  Array/1 -> Assignment/1

== system system_2022 [23-03-03]/Subsystem/Motor Controller/Subsystem ==
  note: limited(22)
  note: Open system conversion factor
      | placed in Pressure Sub-System
  input : Inport
  Prs : Inport  Port=2
  PID Controller : slpidlib/PID Controller  Controller=PID  Form=Parallel  TimeDomain=Continuous-time  UseExternalTs=off  SampleTime=-1  IntegratorMethod=Forward Euler  FilterMethod=Forward Euler  ControllerParametersSource=internal  P=2.39  I=4.49  UseKiTs=off  D=0  N=100  UseFilter=on  TunerSelectOption=Transfer Function Based (PID Tuner App)  InitialConditionSource=internal  InitialConditionForIntegrator=0  InitialConditionForFilter=0  DifferentiatorICPrevScaledInput=0  ExternalReset=none  TrackingMode=off  Kt=1  LimitOutput=off  SatLimitsSource=internal  UpperSaturationLimit=22  LowerSaturationLimit=0  LinearizeAsGain=on  AntiWindupMode=none  Kb=1  POutMin=[]  POutMax=[]  IOutMin=[]  IOutMax=[]  DOutMin=[]  DOutMax=[]  NOutMin=[]  NOutMax=[]  SumOutMin=[]  SumOutMax=[]  SaturationOutMin=[]  SaturationOutMax=[]  PParamMin=[]  PParamMax=[]  IParamMin=[]  IParamMax=[]  DParamMin=[]  DParamMax=[]  NParamMin=[]  NParamMax=[]  KbParamMin=[]  KbParamMax=[]  KtParamMin=[]  KtParamMax=[]  KbOutMin=[]  KbOutMax=[]  KtOutMin=[]  KtOutMax=[]  IntegratorOutMin=[]  IntegratorOutMax=[]  FilterOutMin=[]  FilterOutMax=[]  SumI1OutMin=[]  SumI1OutMax=[]  SumI2OutMin=[]  SumI2OutMax=[]  SumI3OutMin=[]  SumI3OutMax=[]  SumI4OutMin=[]  SumI4OutMax=[]  SumDOutMin=[]  SumDOutMax=[]  DifferentiatorOutMin=[]  DifferentiatorOutMax=[]  FilterDiffOutCoefMin=[]  FilterDiffOutCoefMax=[]  ReciprocalOutMin=[]  ReciprocalOutMax=[]  SumDenOutMin=[]  SumDenOutMax=[]  SumNumOutMin=[]  SumNumOutMax=[]  DivideOutMin=[]  DivideOutMax=[]  UdiffTsProdOutMin=[]  UdiffTsProdOutMax=[]  NTsProdOutMin=[]  NTsProdOutMax=[]  UintegralTsProdOutMin=[]  UintegralTsProdOutMax=[]  UngainTsProdOutMin=[]  UngainTsProdOutMax=[]  IntegratorContinuousStateAttributes=''  IntegratorStateMustResolveToSignalObject=off  IntegratorRTWStateStorageClass=Auto  FilterContinuousStateAttributes=''  FilterStateMustResolveToSignalObject=off  FilterRTWStateStorageClass=Auto  ParallelPVariant=InternalParameters  IdealPVariant=Disabled  IVariant=InternalParameters  DVariant=InternalParameters  IntegratorVariant=Continuous  SatVariant=Disabled  AWVariant=Passthrough  PCopyVariant=Disabled  TRVariant=Disabled  FdbkBlocksVariant=Forward  IdealPFdbkVariant=Disabled  SatFdbkVariant=Disabled  DerivativeFilterVariant=ContFilter  NVariant=InternalParameters  NCopyVariant=Disabled  FilterICVariant=InternalICsFilter  IntegratorICVariant=InternalICs  ExternalResetVariant=Disabled  TRSumVariant=Passthrough  SumFdbkVariant=Disabled  SumVariant=Sum_PID  TsampFilterVariant=InternalTs  TsampNgainVariant=Passthrough  TsampIntegralVariant=Passthrough  ExternalSaturationOutDataTypeStr=Inherit: Same as second input  aMode=0
  Scope : Scope  NumInputPorts=3
  Sum : Sum  Inputs=|+-
  m^3/s to I2C : Gain  Gain=11.5
  PID : Outport
  wires:
  PID Controller/1 -> m^3/s to I2C/1  "PID"
  input/1 -> Scope/2, Sum/1  "mtr_factor"
  m^3/s to I2C/1 -> PID/1
  Sum/1 -> Scope/1, PID Controller/1  "Error"
  Prs/1 -> Sum/2, Scope/3  "prs_factor"

== system system_2022 [23-03-03]/Subsystem/Motor Controller/Subsystem1 ==
  note: limited(22)
  note: Open system conversion factor
      | placed in Pressure Sub-System
  input : Inport
  Prs : Inport  Port=2
  PID Controller : slpidlib/PID Controller  Controller=PID  Form=Parallel  TimeDomain=Continuous-time  UseExternalTs=off  SampleTime=-1  IntegratorMethod=Forward Euler  FilterMethod=Forward Euler  ControllerParametersSource=internal  P=2.39  I=4.49  UseKiTs=off  D=0  N=100  UseFilter=on  TunerSelectOption=Transfer Function Based (PID Tuner App)  InitialConditionSource=internal  InitialConditionForIntegrator=0  InitialConditionForFilter=0  DifferentiatorICPrevScaledInput=0  ExternalReset=none  TrackingMode=off  Kt=1  LimitOutput=off  SatLimitsSource=internal  UpperSaturationLimit=22  LowerSaturationLimit=0  LinearizeAsGain=on  AntiWindupMode=none  Kb=1  POutMin=[]  POutMax=[]  IOutMin=[]  IOutMax=[]  DOutMin=[]  DOutMax=[]  NOutMin=[]  NOutMax=[]  SumOutMin=[]  SumOutMax=[]  SaturationOutMin=[]  SaturationOutMax=[]  PParamMin=[]  PParamMax=[]  IParamMin=[]  IParamMax=[]  DParamMin=[]  DParamMax=[]  NParamMin=[]  NParamMax=[]  KbParamMin=[]  KbParamMax=[]  KtParamMin=[]  KtParamMax=[]  KbOutMin=[]  KbOutMax=[]  KtOutMin=[]  KtOutMax=[]  IntegratorOutMin=[]  IntegratorOutMax=[]  FilterOutMin=[]  FilterOutMax=[]  SumI1OutMin=[]  SumI1OutMax=[]  SumI2OutMin=[]  SumI2OutMax=[]  SumI3OutMin=[]  SumI3OutMax=[]  SumI4OutMin=[]  SumI4OutMax=[]  SumDOutMin=[]  SumDOutMax=[]  DifferentiatorOutMin=[]  DifferentiatorOutMax=[]  FilterDiffOutCoefMin=[]  FilterDiffOutCoefMax=[]  ReciprocalOutMin=[]  ReciprocalOutMax=[]  SumDenOutMin=[]  SumDenOutMax=[]  SumNumOutMin=[]  SumNumOutMax=[]  DivideOutMin=[]  DivideOutMax=[]  UdiffTsProdOutMin=[]  UdiffTsProdOutMax=[]  NTsProdOutMin=[]  NTsProdOutMax=[]  UintegralTsProdOutMin=[]  UintegralTsProdOutMax=[]  UngainTsProdOutMin=[]  UngainTsProdOutMax=[]  IntegratorContinuousStateAttributes=''  IntegratorStateMustResolveToSignalObject=off  IntegratorRTWStateStorageClass=Auto  FilterContinuousStateAttributes=''  FilterStateMustResolveToSignalObject=off  FilterRTWStateStorageClass=Auto  ParallelPVariant=InternalParameters  IdealPVariant=Disabled  IVariant=InternalParameters  DVariant=InternalParameters  IntegratorVariant=Continuous  SatVariant=Disabled  AWVariant=Passthrough  PCopyVariant=Disabled  TRVariant=Disabled  FdbkBlocksVariant=Forward  IdealPFdbkVariant=Disabled  SatFdbkVariant=Disabled  DerivativeFilterVariant=ContFilter  NVariant=InternalParameters  NCopyVariant=Disabled  FilterICVariant=InternalICsFilter  IntegratorICVariant=InternalICs  ExternalResetVariant=Disabled  TRSumVariant=Passthrough  SumFdbkVariant=Disabled  SumVariant=Sum_PID  TsampFilterVariant=InternalTs  TsampNgainVariant=Passthrough  TsampIntegralVariant=Passthrough  ExternalSaturationOutDataTypeStr=Inherit: Same as second input  aMode=0
  Scale(0-1)a : Gain  Gain=0.045
  Scale(0-1)b : Gain  Gain=0.045
  Sum : Sum  Inputs=|+-
  m^3/s to I2C : Gain  Gain=255
  PID : Outport
  wires:
  input/1 -> Scale(0-1)b/1
  PID Controller/1 -> m^3/s to I2C/1  "PID"
  Scale(0-1)b/1 -> Sum/1  "mtr_factor"
  m^3/s to I2C/1 -> PID/1
  Sum/1 -> PID Controller/1  "Error"
  Scale(0-1)a/1 -> Sum/2  "prs_factor"
  Prs/1 -> Scale(0-1)a/1  "prs_factor"

== system system_2022 [23-03-03]/Subsystem/Pressure_Sensor_1/Open System Conversion ==
  note: Conversion Factor for Open Pressure System
      | ( remove once full system is assembled )
  Pressure : Inport
  Add : Sum
  Constant : Constant
  Gain : Gain  Gain=3.75
  Pressure1 : Outport
  wires:
  Add/1 -> Gain/1
  Constant/1 -> Add/2
  Pressure/1 -> Add/1
  Gain/1 -> Pressure1/1
